simulink model "batteryModel"  (R2022b)
settings: Solver=VariableStepAuto  StartTime=0.0  StopTime=80000  RelTol=1e-3
PreLoadFcn:
  | first_run_this_to_import_nedc_data
  | batteryModel_ini
InitFcn:
  | first_run_this_to_import_nedc_data
  | batteryModel_ini
values from neighbouring files (symbols this model uses):
  Battery =     [BatteryParameters.mat]
  I = [1.29210780767e-28 1.29210780767e-28 1.29210780767e-28 1.29210780767e-28 1.29210780767e-28 1.29210780767e-28 1.29210780767e-28 1.29210780767e-28 1.29210780767e-28 1.29210780767e-28 1.29210780767e-28 4.77614030937 ... (41369 elements, 41369x1)]    [BatteryParameters.mat]
  OCVSOC = [2 2 0.95 1.1 0.95 0.79 1.02 0.92 0.75 0.87]    [BatteryParameters.mat]    (also in OCVSOC.mat)
  Ts = 1    [BatteryParameters.mat]    (also in myFunction.m; test1.m)
undefined symbols (not defined in the file or in its folder): sigbuilder_block
libraries: neural x50, fl_lib x7, nesl_utility x6, dspstat3 x3, simulink x2, sharedTrackingLibrary x2, batteryecm_lib x1, ctrlSharedLib x1
(part 1 of 3)
settings Model: Creator=The MathWorks, Inc.  LastModifiedBy=99661217
settings SolverCC: AlgebraicLoopSolver=TrustRegion
settings DataIOCC: SignalLogging=off  DSMLogging=off
settings OptimizationCC: DefaultParameterBehavior=Inlined  EnhancedBackFolding=on  PassReuseOutputArgsAs=Individual arguments  OptimizeBlockOrder=speed  DifferentSizesBufferReuse=on  OptimizationCustomize=off  EfficientTunableParamExpr=on
settings DebuggingCC: ParameterTunabilityLossMsg=error  UnconnectedInputMsg=warning  UnconnectedOutputMsg=warning  UnconnectedLineMsg=warning  PregeneratedLibrarySubsystemCodeDiagnostic=none  SFMachineParentedDataDiag=warning  ArithmeticOperatorsInVariantConditions=warning
settings ModelReferenceCC: EnableRefExpFcnMdlSchedulingChecks=on
settings SFSimCC: SimUseLocalCustomCode=off  MATLABDynamicMemAlloc=off  CustomCodeUndefinedFunction=UseInterfaceOnly
settings RTWCC: Description=Embedded Coder  SystemTargetFile=ert.tlc  GenCodeOnly=on  TemplateMakefile=ert_default_tmf  GenerateReport=on  RTWUseLocalCustomCode=off  IncludeHyperlinkInReport=on  LaunchReport=on  GenerateTraceInfo=on  GenerateTraceReport=on  GenerateTraceReportSl=on  GenerateTraceReportSf=on  GenerateTraceReportEml=on
settings CodeAppCC: ForceParamTrailComments=on  IgnoreCustomStorageClasses=off  OperatorAnnotations=on  SimulinkDataObjDesc=on  SFDataObjDesc=on  InsertBlockDesc=on
settings ERTTargetCC: TargetLangStandard=C99 (ISO)  GenerateSampleERTMain=on  InlinedParameterPlacement=NonHierarchical  ERTCustomFileTemplate=example_file_process.tlc
settings SimscapeCC: SimscapeNormalizeSystem=off

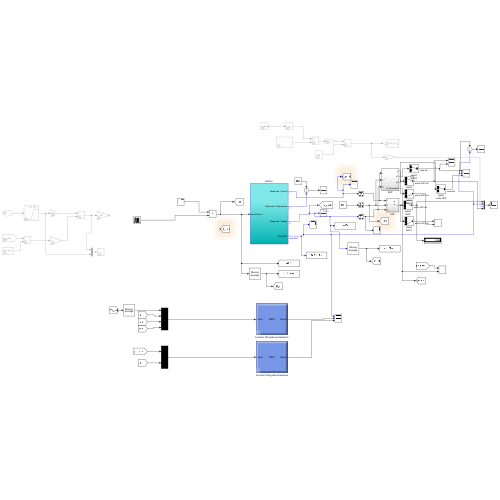
[thumbnail: Simulink's stored preview of the top-level diagram]
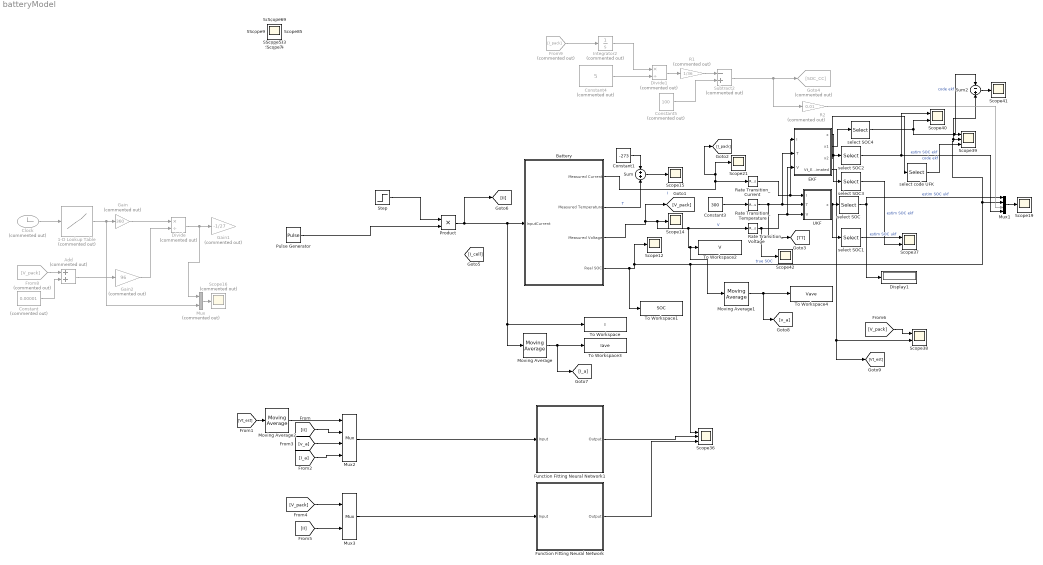
== system batteryModel ==
  1-D Lookup Table : Lookup_n-D  Commented=on  NumberOfTableDimensions=1  BreakpointsForDimension1=t  Table=I  InternalRulePriority=Speed  RndMeth=Simplest
  Add : Sum  Commented=on
  Battery : Subsystem
  Clock : Clock  Commented=on
  Constant : Constant  Commented=on  Value=0.00001
  Constant1 : Constant  Value=-273
  Constant3 : Constant  Value=300
  Constant4 : Constant  Commented=on  Value=5
  Constant5 : Constant  Commented=on  Value=100
  Display1 : Display
  Divide : Product  Commented=on  Inputs=*/
  Divide1 : Product  Commented=on  Inputs=*/
  EKF : Subsystem
  From8 : From  Commented=on  GotoTag=V_pack
  From9 : From  Commented=on  GotoTag=I_pack
  Function Fitting Neural Network : Subsystem
      mask help: Function Fitting Neural Network
      mask Display: e = 0.06;c1 = [120 150 230]/255;c2 = ([120 150 230]+0)/383;c3 = ([120 150 230]+128)/383;patch([0 1 1 0],[0 0 1 1],c1);patch([0 1 1 1-e 1-e 0+e],[0 0 1 1-e 0+e 0+e],c2);patch([0 0 1 1-e 0+e 0+e],[0 1 1 1-e 1-e 0+e],c3);plot([0 1 1 0 0],[0 0 1 1 0]);fprintf('NNET');port_label('input',1,' Input');port_label('output',1,'Output ');
  Function Fitting Neural Network1 : Subsystem
      mask help: Function Fitting Neural Network
      mask Display: e = 0.06;c1 = [120 150 230]/255;c2 = ([120 150 230]+0)/383;c3 = ([120 150 230]+128)/383;patch([0 1 1 0],[0 0 1 1],c1);patch([0 1 1 1-e 1-e 0+e],[0 0 1 1-e 0+e 0+e],c2);patch([0 0 1 1-e 0+e 0+e],[0 1 1 1-e 1-e 0+e],c3);plot([0 1 1 0 0],[0 0 1 1 0]);fprintf('NNET');port_label('input',1,' Input');port_label('output',1,'Output ');
  Gain : Gain  Commented=on  Gain=360
  Gain1 : Gain  Commented=on  Gain=-1/27
  Gain2 : Gain  Commented=on  Gain=96
  Goto4 : Goto  Commented=on  GotoTag=SOC_CC
  Integrator2 : Integrator  Commented=on
  Moving Average : dspstat3/Moving Average  Method=Sliding window  ForgettingFactorPort=off  SpecifyWindowLength=on  WindowLength=10  OverlapLength=9  AllowArbitraryInputLength=off  ForgettingFactor=0.9  SimulateUsing=Code generation
  Moving Average1 : dspstat3/Moving Average  Method=Sliding window  ForgettingFactorPort=off  SpecifyWindowLength=on  WindowLength=10  OverlapLength=9  AllowArbitraryInputLength=off  ForgettingFactor=0.9  SimulateUsing=Code generation
  Moving Average2 : dspstat3/Moving Average  Method=Sliding window  ForgettingFactorPort=off  SpecifyWindowLength=on  WindowLength=10  OverlapLength=9  AllowArbitraryInputLength=off  ForgettingFactor=0.9  SimulateUsing=Code generation
  Mux : Mux  Commented=on  Inputs=2
  Mux1 : Mux
  Mux2 : Mux
  Mux3 : Mux  Inputs=2
  Product : Product
  Pulse Generator : DiscretePulseGenerator  PulseType=Time based  Amplitude=-5  Period=60*60  PulseWidth=5/60*100
  R1 : Gain  Commented=on  Gain=1/36
  R2 : Gain  Commented=on  Gain=0.01
  Rate Transition_Current : RateTransition  OutPortSampleTime=Ts
  Rate Transition_Temperature : RateTransition  InitialCondition=300  OutPortSampleTime=Ts
  Rate Transition_Voltage : RateTransition  InitialCondition=4  OutPortSampleTime=Ts
  Scope{,1..15,17..35,41..42} (37 alike) : Scope
  Scope16 : Scope  Commented=on
  Scope36 : Scope  NumInputPorts=3
  Scope37 : Scope  NumInputPorts=2
  Scope38 : Scope  NumInputPorts=2
  Scope39 : Scope  NumInputPorts=3
  Scope40 : Scope  NumInputPorts=2
  Step : Step  SampleTime=0
  Subtract2 : Sum  Commented=on  Inputs=-+
  Sum : Sum
  Sum2 : Sum  Inputs=-+
  To Workspace : ToWorkspace  VariableName=I  SampleTime=-1
  To Workspace1 : ToWorkspace  VariableName=SOC  SampleTime=-1
  To Workspace2 : ToWorkspace  VariableName=V  SampleTime=-1
  To Workspace3 : ToWorkspace  VariableName=Iave  SampleTime=-1
  To Workspace4 : ToWorkspace  VariableName=Vave  SampleTime=-1
  UKF : Subsystem
  select SOC : Selector  InputPortWidth=5  IndexOptions=Index vector (dialog)  Indices=1  OutputSizes=1
  select SOC1 : Selector  InputPortWidth=5  IndexOptions=Index vector (dialog)  Indices=5  OutputSizes=1
  select SOC2 : Selector  InputPortWidth=5  IndexOptions=Index vector (dialog)  Indices=1  OutputSizes=1
  select SOC3 : Selector  InputPortWidth=5  IndexOptions=Index vector (dialog)  Indices=5  OutputSizes=1
  select SOC4 : Selector  InputPortWidth=2  IndexOptions=Index vector (dialog)  Indices=1  OutputSizes=1
  select code UFK : Selector  InputPortWidth=2  IndexOptions=Index vector (dialog)  Indices=1  OutputSizes=1
  wires:
  Battery/4(Real SOC) -> To Workspace1/1, Scope12/1, Sum2/2, Scope39/2, Mux1/2, Scope36/1  "true SOC"
  Divide/1 -> Gain1/1, Mux/1
  Battery/3(Measured Voltage) -> [V_pack], Moving Average1/1, To Workspace2/1, Rate Transition_Voltage/1, Scope14/1  "V"
  Battery/2(Measured Temperature) -> Sum/2  "T"
  Sum/1 -> Scope15/1
  Constant1/1 -> Sum/1
  From8/1 -> Add/1
  Clock/1 -> 1-D Lookup Table/1
  1-D Lookup Table/1 -> Mux/2, Gain/1
  Mux/1 -> Scope16/1
  Constant/1 -> Add/2
  Gain/1 -> Divide/1
  Add/1 -> Gain2/1
  Gain2/1 -> Divide/2
  Rate Transition_Temperature/1 -> [TT], UKF/2(T), EKF/2(T)
  Rate Transition_Voltage/1 -> Scope42/1, UKF/3(V), EKF/3(V)
  UKF/1(x) -> select SOC1/1, select SOC/1
  Rate Transition_Current/1 -> EKF/1(I), UKF/1(I)
  Battery/1(Measured Current) -> [I_pack], Scope21/1, Rate Transition_Current/1  "I"
  Mux1/1 -> Scope19/1
  select SOC/1 -> Mux1/1, Display1/1  "estim SOC ukf"
  Divide1/1 -> R1/1
  Integrator2/1 -> Divide1/1
  Constant5/1 -> Subtract2/2
  Constant4/1 -> Divide1/2
  R1/1 -> Subtract2/1
  Subtract2/1 -> R2/1, Goto4/1
  From9/1 -> Integrator2/1
  R2/1 -> Mux1/3
  Step/1 -> Product/1
  Product/1 -> [II], Moving Average/1, To Workspace/1, Battery/1(InputCurrent)
  select SOC1/1 -> Scope37/1  "estim SOC ukf"
  Constant3/1 -> Rate Transition_Temperature/1
  EKF/1(x) -> select SOC3/1, select SOC2/1
  select SOC2/1 -> Scope40/1, Mux1/4  "estim SOC ekf"
  select SOC3/1 -> Scope37/2  "estim SOC ekf"
  EKF/2(x1) -> select SOC4/1
  select SOC4/1 -> Sum2/1, Scope39/1, Scope40/2  "code ekf"
  Sum2/1 -> Scope41/1
  EKF/3(x2) -> select code UFK/1
  select code UFK/1 -> Scope39/3  "code ekf"
  Moving Average/1 -> [I_a], To Workspace3/1
  Moving Average1/1 -> [v_a], To Workspace4/1
  Function Fitting Neural Network1/1(Output) -> Scope36/2
  [Vt_est] -> Moving Average2/1
  [II] -> Mux2/2
  [v_a] -> Mux2/3
  [I_a] -> Mux2/4
  Mux2/1 -> Function Fitting Neural Network1/1(Input)
  Function Fitting Neural Network/1(Output) -> Scope36/3
  [V_pack] -> Mux3/1
  [II] -> Mux3/2
  Mux3/1 -> Function Fitting Neural Network/1(Input)
  [V_pack] -> Scope38/1
  EKF/4(Vt_Estimated) -> [Vt_est], Scope38/2
  Moving Average2/1 -> Mux2/1
  Pulse Generator/1 -> Product/2

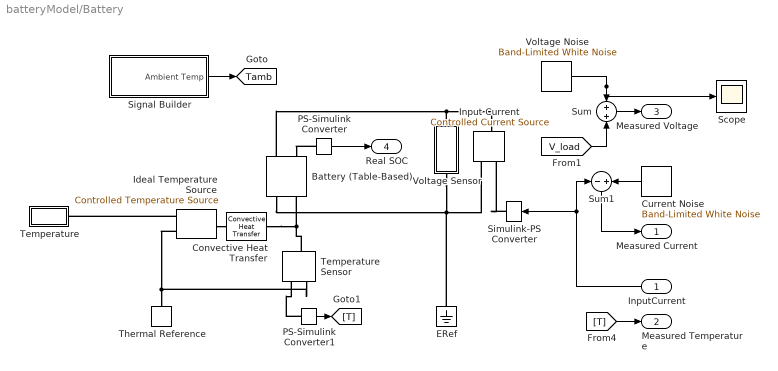
== system batteryModel/Battery ==
  InputCurrent : Inport
  Battery (Table-Based) : batteryecm_lib/Battery (Table-Based)  SOC_vec=Battery(1).SOC_LUT  T_dependence=simscape.enum.tablebattery.temperature_dependence.yes  prm_dir=simscape.enum.tablebattery.prm_dir.noCurrentDirectionality  T_vec=Battery(1).Temperature_LUT K  V0_mat=Battery(1).Em_LUT V  V0_vec=[3.1, 3.27, 3.31, 3.5] V  V_range=[0, inf] V  R0_mat=Battery(1).R0_LUT Ohm  R0_vec=[.015, .017, .012, .013] Ohm  R0_dis_mat=[.0117, .0085, .009; .011, .0085, .009; .0114, .0087, .0092; .0107, .0082, .0088; .0107, .0083, .0091; .0113, .0085, .0089; .0116, .0085, .0089] Ohm  R0_dis_vec=[.0085, .0085, .0087, .0082, .0083, .0085, .0085] Ohm  R0_ch_mat=[.0117, .0085, .009; .011, .0085, .009; .0114, .0087, .0092; .0107, .0082, .0088; .0107, .0083, .0091; .0113, .0085, .0089; .0116, .0085, .0089] Ohm  R0_ch_vec=[.0085, .0085, .0087, .0082, .0083, .0085, .0085] Ohm  AH=Battery(1).Capacity_LUT hr*A  prm_leak=simscape.enum.tablebattery.prm_leak.disabled  Rleak_vec=[8000, 7000, 6000] Ohm  Rleak=7e3 Ohm  extrapolation_option=simscape.enum.extrapolation.linear  SOC_port=simscape.enum.tablebattery.enable.yes  prm_dyn=simscape.enum.tablebattery.prm_dyn.rc3  R1_mat=Battery(1).R1_LUT Ohm  R1_vec=[.076, .022, .007, .043] Ohm  tau1_mat=Battery(1).t1_LUT s  tau1_vec=[148, 110, 27, 22] s  R2_mat=Battery(1).R2_LUT Ohm  R2_vec=[.382, .006, .007, .956] Ohm  tau2_mat=Battery(1).t2_LUT s  tau2_vec=[44, 24, 14, 13419] s  R3_mat=Battery(1).R3_LUT Ohm  R3_vec=[.382, .006, .007, .956] Ohm  tau3_mat=Battery(1).t3_LUT s  tau3_vec=[44, 24, 14, 13419] s  R4_mat=[.014, .382, .407; .028, .006, .007; .014, .007, .006; .333, .956, .912] Ohm  R4_vec=[.382, .006, .007, .956] Ohm  tau4_mat=[1, 44, 5644; 11, 24, 506; 2, 14, 330; 3310, 13419, 30216] s  tau4_vec=[44, 24, 14, 13419] s  R5_mat=[.014, .382, .407; .028, .006, .007; .014, .007, .006; .333, .956, .912] Ohm  R5_vec=[.382, .006, .007, .956] Ohm  tau5_mat=[1, 44, 5644; 11, 24, 506; 2, 14, 330; 3310, 13419, 30216] s  tau5_vec=[44, 24, 14, 13419] s  prm_fade=simscape.enum.tablebattery.prm_fade.equations  N0=100  dV0=0  dR0=0  dAH=0  dRleak=0  dR1=0  dR2=0  dR3=0  dR4=0  dR5=0  N0vec=[100, 200, 300]  Tfadevec=[298.15, 323.15] K  dV0vec=[0, 0, 0]  dR0vec=[0, 0, 0]  dAHvec=[0, 0, 0]  dRleakvec=[0, 0, 0]  dR1vec=[0, 0, 0]  dR2vec=[0, 0, 0]  dR3vec=[0, 0, 0]  dR4vec=[0, 0, 0]  dR5vec=[0, 0, 0]  dV0mat=[0, 0; 0, 0; 0, 0]  dR0mat=[0, 0; 0, 0; 0, 0]  dAHmat=[0, 0; 0, 0; 0, 0]  dRleakmat=[0, 0; 0, 0; 0, 0]  dR1mat=[0, 0; 0, 0; 0, 0]  dR2mat=[0, 0; 0, 0; 0, 0]  dR3mat=[0, 0; 0, 0; 0, 0]  dR4mat=[0, 0; 0, 0; 0, 0]  dR5mat=[0, 0; 0, 0; 0, 0]  prm_age_modeling=simscape.enum.tablebattery.prm_age_modeling.equation  storage_dt_age_vec=[0] d  storage_T_age_vec=[273] K  prm_age_OCV=simscape.enum.tablebattery.prm_age_OCV.OCV  OCV_age=0.9  SOC_age=0.6  prm_age_resistance=simscape.enum.tablebattery.prm_age.disabled  OCV_scaling_age_resistance=2.2134e6  OCV_offset_age_resistance=1.632e6  temp_exp_age_resistance=0.515833569 V  t_exp_age_resistance=0.75  T_age_vec_resistance=[273.15, 298.15, 323.15] K  dt_age_vec_resistance=[90, 180, 270, 360] d  dR0_age_vec=[0, 0, 0]  t_meas_dR0_age=100 d  dR0_age_mat=[0, 0, 0; 0, 0, 0; 0, 0, 0; 0, 0, 0]  prm_age_capacity=simscape.enum.tablebattery.prm_age.disabled  OCV_scaling_age_capacity=1.5097e07  OCV_offset_age_capacity=8.3625e06  temp_exp_age_capacity=0.6011 V  t_exp_age_capacity=0.75  T_age_vec_capacity=[273.15, 298.15, 323.15] K  dt_age_vec_capacity=[90, 180, 270, 360] d  dAH_age_vec=[0, 0, 0]  t_meas_dAH_age=100 d  dAH_age_mat=[0, 0, 0; 0, 0, 0; 0, 0, 0; 0, 0, 0]  thermal_port=simscape.enum.thermaleffects.model  temperature=Battery(1).T_init K  thermal_mass=Battery(1).cell_Cp_heat * Battery(1).cell_mass J/K  i_specify=off  i_priority=None  i=0 A  i_nominal_specify=off  i_nominal_unit=A  i_nominal_value=1  v_specify=off  v_priority=None  v=0 V  v_nominal_specify=off  v_nominal_unit=V  v_nominal_value=1  stateOfCharge_specify=on  stateOfCharge_priority=High  stateOfCharge=Battery(1).SOC0  stateOfCharge_nominal_specify=off  stateOfCharge_nominal_unit=1  stateOfCharge_nominal_value=1  num_cycles_specify=off  num_cycles_priority=High  num_cycles=0  num_cycles_nominal_specify=off  num_cycles_nominal_unit=1  num_cycles_nominal_value=1  cell_temperature_specify=off  cell_temperature_priority=High  cell_temperature=Battery(1).T_init K  cell_temperature_nominal_specify=off  cell_temperature_nominal_unit=K  cell_temperature_nominal_value=1
  Convective Heat Transfer : fl_lib/Thermal/Thermal Elements/Convective Heat Transfer  thermal_type=foundation.enum.constant_variable.constant  area=cell_area m^2  heat_tr_coeff=h_conv W/(m^2 * K)  min_heat_tr_coeff=1e-3 W/(K*m^2)  T_specify=off  T_priority=High  T=0 K  T_nominal_specify=off  T_nominal_unit=K  T_nominal_value=1  Q_specify=off  Q_priority=High  Q=0 J/s  Q_nominal_specify=off  Q_nominal_unit=J/s  Q_nominal_value=1
  Current Noise : simulink/Sources/Band-Limited White Noise  Cov=2.5e-2  Ts=Ts  seed=[1234]
  ERef : fl_lib/Electrical/Electrical Elements/Electrical Reference
  Ideal Temperature Source : fl_lib/Thermal/Thermal Sources/Controlled Temperature Source
  Input Current : fl_lib/Electrical/Electrical Sources/Controlled Current Source
  PS-Simulink Converter : nesl_utility/PS-Simulink Converter  PhysicalDomain=network_engine_domain  SubClassName=ps_output  LeftPortType=input  RightPortType=output  PseudoPeriodic=off  Frequencies=[]  VectorFormat=1-D array  Unit=inherit  AffineConversion=off
  PS-Simulink Converter1 : nesl_utility/PS-Simulink Converter  PhysicalDomain=network_engine_domain  SubClassName=ps_output  LeftPortType=input  RightPortType=output  PseudoPeriodic=off  Frequencies=[]  VectorFormat=1-D array  Unit=inherit  AffineConversion=off
  Scope : Scope
  Signal Builder : Subsystem  Tag=STV Subsys  LoadFcn=sigbuilder_block('load');  StartFcn=sigbuilder_block('start');  StopFcn=sigbuilder_block('stop');  ClipboardFcn=sigbuilder_block('clipboard');  mask(Sigbuilder block){tuvar=[0:10]}
      mask help: Simulink:masks:SigbuilderBlock_MD
      mask init:
      | if ~strcmp(get_param(bdroot(gcbh),'SimulationStatus'),'stopped') tuvar = sigbuilder_block('maskInit'); end
      settings: CopyFcn=sigbuilder_block('copy');  DeleteFcn=sigbuilder_block('delete');  ModelCloseFcn=sigbuilder_block('modelClose');  PreSaveFcn=sigbuilder_block('preSave');  PauseFcn=sigbuilder_block('pause');  ContinueFcn=sigbuilder_block('continue');  NameChangeFcn=sigbuilder_block('namechange');  OpenFcn=sigbuilder_block('open',[45.6 240 978 346.2 ]);  CloseFcn=sigbuilder_block('close');
      mask Display: plot(0, 0, 100, 100,[2, 2, 32, 32, 2], [68, 8, 8, 68, 68],[32, 2], [38, 38], [32, 19, 2],[53, 60, 44], [32, 17, 17, 2],[16, 16, 31, 31]);txt = getActiveGroup(gcbh);text(2, 100, txt,'verticalAlignment', 'top');
  Simulink-PS Converter : nesl_utility/Simulink-PS Converter  PhysicalDomain=network_engine_domain  SubClassName=ps_input  LeftPortType=input  RightPortType=output  PseudoPeriodic=off  Frequencies=[]  NoiseDistribution=none  NoiseParameters=[]  Unit=A  AffineConversion=off  FilteringAndDerivatives=zero  SimscapeFilterOrder=1  InputFilterTimeConstant=.001  UdotUserProvided=1
  Sum : Sum
  Sum1 : Sum  Inputs=-+
  Temperature : Subsystem
      mask Display: disp('Tamb')
  Temperature Sensor : fl_lib/Thermal/Thermal Sensors/Temperature Sensor
  Thermal Reference : fl_lib/Thermal/Thermal Elements/Thermal Reference
  Voltage Sensor : Subsystem
      mask Display: disp('V_load')
  Voltage Noise : simulink/Sources/Band-Limited White Noise  Cov=0.5e-3  Ts=Ts  seed=[1234]
  Measured Current : Outport  VectorParamsAs1DForOutWhenUnconnected=off
  Measured Temperature : Outport  Port=2  VectorParamsAs1DForOutWhenUnconnected=off
  Measured Voltage : Outport  Port=3  VectorParamsAs1DForOutWhenUnconnected=off
  Real SOC : Outport  Port=4  VectorParamsAs1DForOutWhenUnconnected=off
  tag scope: Tamb=global
  wires:
  Signal Builder/1(Ambient Temp) -> [Tamb]
  [V_load] -> Sum/2
  Sum/1 -> Measured Voltage/1
  Sum1/1 -> Measured Current/1
  InputCurrent/1 -> Sum1/1, Simulink-PS Converter/1
  [T] -> Measured Temperature/1
  PS-Simulink Converter/1 -> Real SOC/1
  PS-Simulink Converter1/1 -> [T]
  Voltage Noise/1 -> Scope/1, Sum/1
  Current Noise/1 -> Sum1/2
  connections:
  Convective Heat Transfer/RConn1 -- Battery (Table-Based)/RConn2 -- Temperature Sensor/LConn1
  Voltage Sensor/RConn1 -- Input Current/RConn2 -- ERef/LConn1 -- Battery (Table-Based)/RConn1
  Battery (Table-Based)/LConn1 -- Input Current/LConn1 -- Voltage Sensor/LConn1
  Ideal Temperature Source/RConn1 -- Temperature/LConn1
  Ideal Temperature Source/RConn2 -- Thermal Reference/LConn1 -- Temperature Sensor/RConn1
  Simulink-PS Converter/RConn1 -- Input Current/RConn1
  Ideal Temperature Source/LConn1 -- Convective Heat Transfer/LConn1
  PS-Simulink Converter/LConn1 -- Battery (Table-Based)/LConn2
  PS-Simulink Converter1/LConn1 -- Temperature Sensor/RConn2

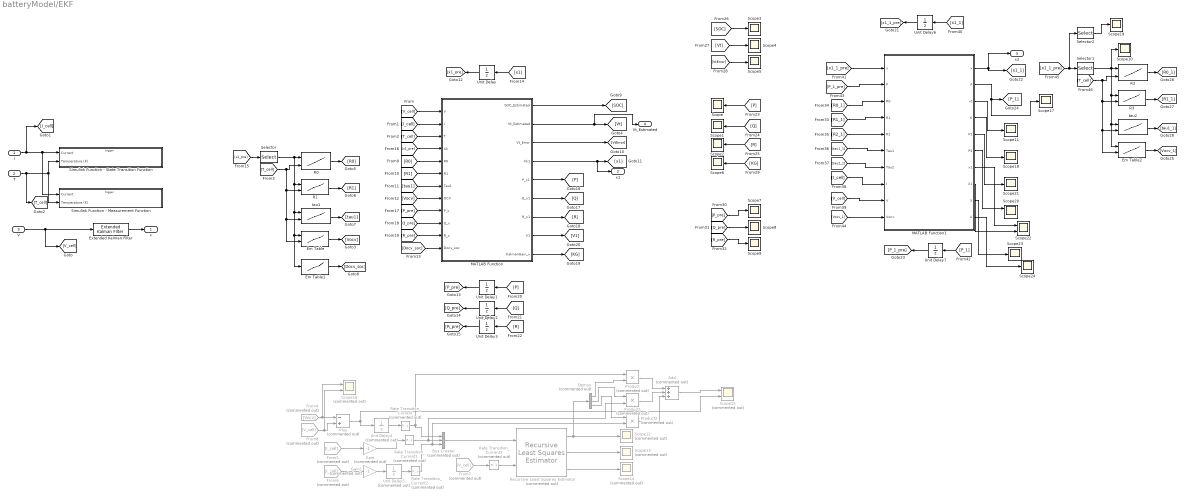
== system batteryModel/EKF ==
  I : Inport
  T : Inport  Port=2
  V : Inport  Port=3
  Add : Sum  Commented=on  Inputs=+++
  Bus Creator : BusCreator  Commented=on  Inputs=3
  Demux : Demux  Commented=on  Outputs=3
  Em Table : Lookup_n-D  BreakpointsForDimension1=Battery.SOC_LUT  BreakpointsForDimension2=Battery.Temperature_LUT  Table=Battery.Em_LUT  InternalRulePriority=Speed  RndMeth=Simplest
      settings: InputPortMap=u0,u1
  Em Table1 : Lookup_n-D  NumberOfTableDimensions=1  BreakpointsForDimension1=Battery.SOC_LUT  BreakpointsForDimension2=Battery.Temperature_LUT  Table=OCVSOC  InternalRulePriority=Speed  RndMeth=Simplest
  Em Table2 : Lookup_n-D  BreakpointsForDimension1=Battery.SOC_LUT  BreakpointsForDimension2=Battery.Temperature_LUT  Table=Battery.Em_LUT  InternalRulePriority=Speed  RndMeth=Simplest
      settings: InputPortMap=u0,u1
  Extended Kalman Filter : sharedTrackingLibrary/Extended Kalman Filter  StateTransitionFcn=batteryStateFcn1  HasStateTransitionJacobianFcn=off  HasAdditiveProcessNoise=Additive  ProcessNoise=1e-10*eye(5)  HasTimeVaryingProcessNoise=off  HasStateTransitionFcnExtraArgument=0  InitialState=[0.1; 0; 0; 0; 0]  InitialStateCovariance=[2000 1 1 1 1]  MeasurementFcn1=batteryMeasurementFcn1  HasMeasurementJacobianFcn1=off  HasMeasurementEnablePort1=off  HasAdditiveMeasurementNoise1=Additive  MeasurementNoise1=50  HasTimeVaryingMeasurementNoise1=off  HasMeasurementFcnExtraArgument1=0  HasMeasurementWrapping1=off  MeasurementFcn2=myMeasurementFcn  HasMeasurementJacobianFcn2=off  HasMeasurementEnablePort2=off  HasAdditiveMeasurementNoise2=Additive  MeasurementNoise2=1  HasTimeVaryingMeasurementNoise2=off  HasMeasurementFcnExtraArgument2=0  HasMeasurementWrapping2=off  MeasurementFcn3=myMeasurementFcn  HasMeasurementJacobianFcn3=off  HasMeasurementEnablePort3=off  HasAdditiveMeasurementNoise3=Additive  MeasurementNoise3=1  HasTimeVaryingMeasurementNoise3=off  HasMeasurementFcnExtraArgument3=0  HasMeasurementWrapping3=off  MeasurementFcn4=myMeasurementFcn  HasMeasurementJacobianFcn4=off  HasMeasurementEnablePort4=off  HasAdditiveMeasurementNoise4=Additive  MeasurementNoise4=1  HasTimeVaryingMeasurementNoise4=off  HasMeasurementFcnExtraArgument4=0  HasMeasurementWrapping4=off  MeasurementFcn5=myMeasurementFcn  HasMeasurementJacobianFcn5=off  HasMeasurementEnablePort5=off  HasAdditiveMeasurementNoise5=Additive  MeasurementNoise5=1  HasTimeVaryingMeasurementNoise5=off  HasMeasurementFcnExtraArgument5=0  HasMeasurementWrapping5=off  EnableMultirate=off  StateTransitionFcnSampleTime=1  MeasurementFcn1SampleTime=1  MeasurementFcn2SampleTime=1  MeasurementFcn3SampleTime=1  MeasurementFcn4SampleTime=1  MeasurementFcn5SampleTime=1  UseCurrentEstimator=off  OutputStateCovariance=off  DataType=double  SampleTime=Ts  NumberOfMeasurements=1
  From4 : From  Commented=on  GotoTag=Vocv
  From5 : From  Commented=on  GotoTag=I_cell
  From6 : From  Commented=on  GotoTag=I_cell
  From7 : From  Commented=on  GotoTag=V_cell
  From8 : From  Commented=on  GotoTag=V_cell
  Gain : Gain  Commented=on  Gain=-1
  Gain1 : Gain  Commented=on  Gain=-1
  MATLAB Function : MATLAB Function  TreatAsAtomicUnit=on
  MATLAB Function1 : MATLAB Function  TreatAsAtomicUnit=on  SystemSampleTime=Ts
  Plus : Sum  Commented=on  Inputs=-+
  Product : Product  Commented=on
  Product1 : Product  Commented=on
  Product2 : Product  Commented=on
  R0 : Lookup_n-D  BreakpointsForDimension1=Battery.SOC_LUT  BreakpointsForDimension2=Battery.Temperature_LUT  Table=Battery.R0_LUT  InternalRulePriority=Speed  RndMeth=Simplest
      settings: InputPortMap=u0,u1
  R1 : Lookup_n-D  BreakpointsForDimension1=Battery.SOC_LUT  BreakpointsForDimension2=Battery.Temperature_LUT  Table=Battery.R1_LUT  InternalRulePriority=Speed  RndMeth=Simplest
      settings: InputPortMap=u0,u1
  R2 : Lookup_n-D  BreakpointsForDimension1=Battery.SOC_LUT  BreakpointsForDimension2=Battery.Temperature_LUT  Table=Battery.R0_LUT  InternalRulePriority=Speed  RndMeth=Simplest
      settings: InputPortMap=u0,u1
  R3 : Lookup_n-D  BreakpointsForDimension1=Battery.SOC_LUT  BreakpointsForDimension2=Battery.Temperature_LUT  Table=Battery.R1_LUT  InternalRulePriority=Speed  RndMeth=Simplest
      settings: InputPortMap=u0,u1
  Rate Transition_Current{,1..3} (4 alike) : RateTransition  Commented=on  OutPortSampleTime=2*Ts
  Recursive Least Squares Estimator : ctrlSharedLib/Recursive Least Squares Estimator  Commented=on  InitialEstimateSource=None  InitialParameterData=3  P0=[1000 0 0;0 1000 0;0 0 1000]  InitialRegressors=0  InitialOutputs=0  History=Infinite  WindowLength=300  EstimationMethod=Forgetting Factor  AdaptationParameter=0.98  HasTimeVaryingAdaptationParameter=off  NormalizationBias=eps  OutputError=on  OutputP=on  AddEnablePort=off  InputProcessing=Sample-based  Ts=2*Ts
      settings: LibrarySourceBlock=slident/Estimators/Recursive Least Squares Estimator
  Scope{,1..11,17..19,21,23..24} (18 alike) : Scope
  Scope12 : Scope  Commented=on
  Scope13 : Scope  Commented=on
  Scope14 : Scope  Commented=on
  Scope15 : Scope  Commented=on  NumInputPorts=2
  Scope16 : Scope  Commented=on  NumInputPorts=2
  Scope20 : Scope  NumInputPorts=2
  Scope22 : Scope  NumInputPorts=2
  Selector : Selector  InputPortWidth=2  IndexOptions=Index vector (dialog)  Indices=[1]  OutputSizes=1
  Selector1 : Selector  InputPortWidth=2  IndexOptions=Index vector (dialog)  Indices=[1]  OutputSizes=1
  Selector2 : Selector  InputPortWidth=2  IndexOptions=Index vector (dialog)  Indices=[2]  OutputSizes=1
  Simulink Function - Measurement Function : Subsystem  TreatAsAtomicUnit=on
  Simulink Function - State Transition Function : Subsystem  TreatAsAtomicUnit=on
  Unit Delay : UnitDelay  InitialCondition=[1 0]  SampleTime=Ts  HasFrameUpgradeWarning=on
  Unit Delay1 : UnitDelay  InitialCondition=[200 0 ;0 1]  SampleTime=Ts  HasFrameUpgradeWarning=on
  Unit Delay2 : UnitDelay  InitialCondition=[1.0e-10 0 ;0 1.0e-10]  SampleTime=Ts  HasFrameUpgradeWarning=on
  Unit Delay3 : UnitDelay  InitialCondition=50  SampleTime=Ts  HasFrameUpgradeWarning=on
  Unit Delay4 : UnitDelay  Commented=on  SampleTime=Ts  HasFrameUpgradeWarning=on
  Unit Delay5 : UnitDelay  Commented=on  SampleTime=Ts  HasFrameUpgradeWarning=on
  Unit Delay6 : UnitDelay  InitialCondition=[1 0]  SampleTime=Ts  HasFrameUpgradeWarning=on
  Unit Delay7 : UnitDelay  InitialCondition=[1 0 ;0 1]  SampleTime=Ts  HasFrameUpgradeWarning=on
  tau1 : Lookup_n-D  BreakpointsForDimension1=Battery.SOC_LUT  BreakpointsForDimension2=Battery.Temperature_LUT  Table=Battery.t1_LUT  InternalRulePriority=Speed  RndMeth=Simplest
      settings: InputPortMap=u0,u1
  tau2 : Lookup_n-D  BreakpointsForDimension1=Battery.SOC_LUT  BreakpointsForDimension2=Battery.Temperature_LUT  Table=Battery.t1_LUT  InternalRulePriority=Speed  RndMeth=Simplest
      settings: InputPortMap=u0,u1
  x : Outport  VectorParamsAs1DForOutWhenUnconnected=off
  x1 : Outport  Port=2  VectorParamsAs1DForOutWhenUnconnected=off
  x2 : Outport  Port=3  VectorParamsAs1DForOutWhenUnconnected=off
  Vt_Estimated : Outport  Port=4
  wires:
  V/1 -> [V_cell], Extended Kalman Filter/1
  T/1 -> [T_cell], Simulink Function - Measurement Function/2(Temperature (K)), Simulink Function - State Transition Function/2(Temperature (K))
  I/1 -> [I_cell], Simulink Function - Measurement Function/1(Current), Simulink Function - State Transition Function/1(Current)
  Extended Kalman Filter/1 -> x/1
  MATLAB Function/4(Xk1) -> [x1], x1/1
  [V_cell] -> MATLAB Function/1(V)
  [I_cell] -> MATLAB Function/2(I)
  [T_cell] -> MATLAB Function/3(T)
  Selector/1 -> Em Table1/1, Em Table/1, tau1/1, R1/1, R0/1
  [T_cell] -> Em Table/2, tau1/2, R1/2, R0/2
  Em Table/1 -> [Vocv]
  MATLAB Function/1(SOC_Estimated) -> [SOC]
  From6/1 -> Gain1/1
  Unit Delay4/1 -> Rate Transition_Current/1
  From5/1 -> Gain/1
  Unit Delay5/1 -> Rate Transition_Current2/1
  Bus Creator/1 -> Recursive Least Squares Estimator/1
  From7/1 -> Rate Transition_Current3/1
  Recursive Least Squares Estimator/1 -> Demux/1, Scope12/1
  From4/1 -> Scope16/1, Plus/1
  From8/1 -> Scope16/2, Plus/2
  Plus/1 -> Scope15/2, Unit Delay4/1
  Gain/1 -> Rate Transition_Current1/1
  Gain1/1 -> Unit Delay5/1
  Recursive Least Squares Estimator/2 -> Scope13/1
  Recursive Least Squares Estimator/3 -> Scope14/1
  Demux/1 -> Product/2
  Demux/2 -> Product1/1
  Demux/3 -> Product2/1
  Product/1 -> Add/1
  Product1/1 -> Add/2
  Product2/1 -> Add/3
  Add/1 -> Scope15/1
  Rate Transition_Current/1 -> Product/1, Bus Creator/1
  Rate Transition_Current1/1 -> Product1/2, Bus Creator/2
  Rate Transition_Current2/1 -> Product2/2, Bus Creator/3
  Rate Transition_Current3/1 -> Recursive Least Squares Estimator/2
  R0/1 -> [R0]
  [R0] -> MATLAB Function/5(R0)
  R1/1 -> [R1]
  [R1] -> MATLAB Function/6(R1)
  tau1/1 -> [tau1]
  [tau1] -> MATLAB Function/7(Tau1)
  Em Table1/1 -> [Docv_soc]
  [Vocv] -> MATLAB Function/8(OCV)
  [Docv_soc] -> MATLAB Function/12(Docv_soc)
  MATLAB Function/2(Vt_Estimated) -> Vt_Estimated/1, [Vt]
  MATLAB Function/3(Vt_Error) -> [VtError]
  [x1] -> Unit Delay/1
  Unit Delay/1 -> [x1_pre]
  [x1_pre] -> Selector/1
  [x1_pre] -> MATLAB Function/4(Xk)
  [P_pre] -> MATLAB Function/9(P_x)
  [Q_pre] -> MATLAB Function/10(Q_x)
  [R_pre] -> MATLAB Function/11(R_x)
  Unit Delay1/1 -> [P_pre]
  Unit Delay2/1 -> [Q_pre]
  Unit Delay3/1 -> [R_pre]
  MATLAB Function/5(P_x1) -> [P]
  MATLAB Function/6(Q_x1) -> [Q]
  MATLAB Function/7(R_x1) -> [R]
  MATLAB Function/9(KalmanGain_x) -> [KG]
  [P] -> Unit Delay1/1
  [Q] -> Unit Delay2/1
  [R] -> Unit Delay3/1
  MATLAB Function/8(V1) -> [V1]
  [P] -> Scope/1
  [Q] -> Scope1/1
  [R] -> Scope2/1
  [SOC] -> Scope3/1
  [Vt] -> Scope4/1
  [VtError] -> Scope5/1
  [KG] -> Scope6/1
  [P_pre] -> Scope7/1
  [Q_pre] -> Scope8/1
  [R_pre] -> Scope9/1
  [R2_1] -> MATLAB Function1/5(R2)
  [R1_1] -> MATLAB Function1/4(R1)
  [R0_1] -> MATLAB Function1/3(R0)
  [tau1_1] -> MATLAB Function1/6(Tau1)
  [tau2_1] -> MATLAB Function1/7(Tau2)
  [I_cell] -> MATLAB Function1/8(I)
  [V_cell] -> MATLAB Function1/9(V)
  Unit Delay6/1 -> [x1_1_pre]
  [x1_1] -> Unit Delay6/1
  MATLAB Function1/1(x) -> [x1_1], x2/1
  [x1_1_pre] -> MATLAB Function1/1("x ")
  Unit Delay7/1 -> [P_1_pre]
  [P_1] -> Unit Delay7/1
  MATLAB Function1/2(P) -> Scope17/1, [P_1]
  [P_1_pre] -> MATLAB Function1/2("P ")
  [Vocv_1] -> MATLAB Function1/10(Vocv)
  [x1_1_pre] -> Selector2/1, Selector1/1
  tau2/1 -> [tau1_1]
  R3/1 -> [R1_1]
  R2/1 -> [R0_1]
  Em Table2/1 -> [Vocv_1]
  [T_cell] -> R2/2, R3/2, tau2/2, Em Table2/2
  Selector1/1 -> Scope10/1, R2/1, R3/1, tau2/1, Em Table2/1
  MATLAB Function1/3(vt) -> Scope11/1
  MATLAB Function1/4(K) -> Scope18/1
  Selector2/1 -> Scope19/1
  MATLAB Function1/6(P2) -> Scope20/1
  MATLAB Function1/5(P1) -> Scope21/1
  MATLAB Function1/7(x1) -> Scope22/1
  MATLAB Function1/8(X1) -> Scope22/2
  MATLAB Function1/9(X) -> Scope23/1
  MATLAB Function1/10(A) -> Scope24/1

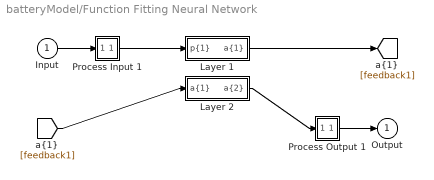
== system batteryModel/Function Fitting Neural Network ==
  Input : Inport  PortDimensions=2
      mask Display: e = 0.06;c1 = [120 230 180]/255;c2 = ([120 230 180]+0)/(256+128);c3 = ([120 230 180]+128)/(256+128);patch([0 1 1 0],[0 0 1 1],c1);patch([0 1 1 1-e 1-e 0+e],[0 0 1 1-e 0+e 0+e],c2);patch([0 0 1 1-e 0+e 0+e],[0 1 1 1-e 1-e 0+e],c3);plot([0 1 1 0 0],[0 0 1 1 0]);
  Layer 1 : Subsystem
      mask Display: e = 0.06;c1 = [120 150 230]/255;c2 = ([120 150 230]+0)/383;c3 = ([120 150 230]+128)/383;patch([0 1 1 0],[0 0 1 1],c1);patch([0 1 1 1-e 1-e 0+e],[0 0 1 1-e 0+e 0+e],c2);patch([0 0 1 1-e 0+e 0+e],[0 1 1 1-e 1-e 0+e],c3);plot([0 1 1 0 0],[0 0 1 1 0]);
  Layer 2 : Subsystem
      mask Display: e = 0.06;c1 = [120 150 230]/255;c2 = ([120 150 230]+0)/383;c3 = ([120 150 230]+128)/383;patch([0 1 1 0],[0 0 1 1],c1);patch([0 1 1 1-e 1-e 0+e],[0 0 1 1-e 0+e 0+e],c2);patch([0 0 1 1-e 0+e 0+e],[0 1 1 1-e 1-e 0+e],c3);plot([0 1 1 0 0],[0 0 1 1 0]);
  Process Input 1 : Subsystem
      mask Display: e = 0.06;c1 = [120 150 230]/255;c2 = ([120 150 230]+0)/383;c3 = ([120 150 230]+128)/383;patch([0 1 1 0],[0 0 1 1],c1);patch([0 1 1 1-e 1-e 0+e],[0 0 1 1-e 0+e 0+e],c2);patch([0 0 1 1-e 0+e 0+e],[0 1 1 1-e 1-e 0+e],c3);plot([0 1 1 0 0],[0 0 1 1 0]);
  Process Output 1 : Subsystem
      mask Display: e = 0.06;c1 = [120 150 230]/255;c2 = ([120 150 230]+0)/383;c3 = ([120 150 230]+128)/383;patch([0 1 1 0],[0 0 1 1],c1);patch([0 1 1 1-e 1-e 0+e],[0 0 1 1-e 0+e 0+e],c2);patch([0 0 1 1-e 0+e 0+e],[0 1 1 1-e 1-e 0+e],c3);plot([0 1 1 0 0],[0 0 1 1 0]);
  Output : Outport  InitialOutput=0
      mask Display: e = 0.06;c1 = [120 230 180]/255;c2 = ([120 230 180]+0)/(256+128);c3 = ([120 230 180]+128)/(256+128);patch([0 1 1 0],[0 0 1 1],c1);patch([0 1 1 1-e 1-e 0+e],[0 0 1 1-e 0+e 0+e],c2);patch([0 0 1 1-e 0+e 0+e],[0 1 1 1-e 1-e 0+e],c3);plot([0 1 1 0 0],[0 0 1 1 0]);
  wires:
  Input/1 -> Process Input 1/1(x)
  Process Output 1/1(y) -> Output/1
  Process Input 1/1(p) -> Layer 1/1("p{1}")
  Layer 1/1("a{1}") -> [feedback1]
  [feedback1] -> Layer 2/1("a{1} ")
  Layer 2/1("a{2}") -> Process Output 1/1(a)

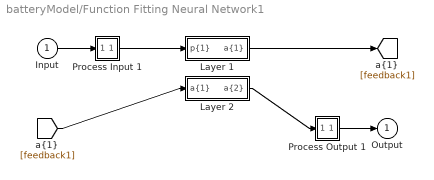
== system batteryModel/Function Fitting Neural Network1 ==
  Input : Inport  PortDimensions=4
      mask Display: e = 0.06;c1 = [120 230 180]/255;c2 = ([120 230 180]+0)/(256+128);c3 = ([120 230 180]+128)/(256+128);patch([0 1 1 0],[0 0 1 1],c1);patch([0 1 1 1-e 1-e 0+e],[0 0 1 1-e 0+e 0+e],c2);patch([0 0 1 1-e 0+e 0+e],[0 1 1 1-e 1-e 0+e],c3);plot([0 1 1 0 0],[0 0 1 1 0]);
  Layer 1 : Subsystem
      mask Display: e = 0.06;c1 = [120 150 230]/255;c2 = ([120 150 230]+0)/383;c3 = ([120 150 230]+128)/383;patch([0 1 1 0],[0 0 1 1],c1);patch([0 1 1 1-e 1-e 0+e],[0 0 1 1-e 0+e 0+e],c2);patch([0 0 1 1-e 0+e 0+e],[0 1 1 1-e 1-e 0+e],c3);plot([0 1 1 0 0],[0 0 1 1 0]);
  Layer 2 : Subsystem
      mask Display: e = 0.06;c1 = [120 150 230]/255;c2 = ([120 150 230]+0)/383;c3 = ([120 150 230]+128)/383;patch([0 1 1 0],[0 0 1 1],c1);patch([0 1 1 1-e 1-e 0+e],[0 0 1 1-e 0+e 0+e],c2);patch([0 0 1 1-e 0+e 0+e],[0 1 1 1-e 1-e 0+e],c3);plot([0 1 1 0 0],[0 0 1 1 0]);
  Process Input 1 : Subsystem
      mask Display: e = 0.06;c1 = [120 150 230]/255;c2 = ([120 150 230]+0)/383;c3 = ([120 150 230]+128)/383;patch([0 1 1 0],[0 0 1 1],c1);patch([0 1 1 1-e 1-e 0+e],[0 0 1 1-e 0+e 0+e],c2);patch([0 0 1 1-e 0+e 0+e],[0 1 1 1-e 1-e 0+e],c3);plot([0 1 1 0 0],[0 0 1 1 0]);
  Process Output 1 : Subsystem
      mask Display: e = 0.06;c1 = [120 150 230]/255;c2 = ([120 150 230]+0)/383;c3 = ([120 150 230]+128)/383;patch([0 1 1 0],[0 0 1 1],c1);patch([0 1 1 1-e 1-e 0+e],[0 0 1 1-e 0+e 0+e],c2);patch([0 0 1 1-e 0+e 0+e],[0 1 1 1-e 1-e 0+e],c3);plot([0 1 1 0 0],[0 0 1 1 0]);
  Output : Outport  InitialOutput=0
      mask Display: e = 0.06;c1 = [120 230 180]/255;c2 = ([120 230 180]+0)/(256+128);c3 = ([120 230 180]+128)/(256+128);patch([0 1 1 0],[0 0 1 1],c1);patch([0 1 1 1-e 1-e 0+e],[0 0 1 1-e 0+e 0+e],c2);patch([0 0 1 1-e 0+e 0+e],[0 1 1 1-e 1-e 0+e],c3);plot([0 1 1 0 0],[0 0 1 1 0]);
  wires:
  Input/1 -> Process Input 1/1(x)
  Process Output 1/1(y) -> Output/1
  Process Input 1/1(p) -> Layer 1/1("p{1}")
  Layer 1/1("a{1}") -> [feedback1]
  [feedback1] -> Layer 2/1("a{1} ")
  Layer 2/1("a{2}") -> Process Output 1/1(a)

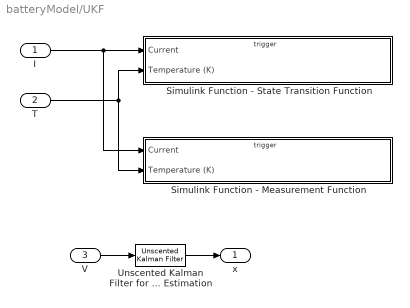
== system batteryModel/UKF ==
  I : Inport
  T : Inport  Port=2
  V : Inport  Port=3
  Simulink Function - Measurement Function : Subsystem  TreatAsAtomicUnit=on
  Simulink Function - State Transition Function : Subsystem  TreatAsAtomicUnit=on
  Unscented Kalman Filter for SOC Estimation : sharedTrackingLibrary/Unscented Kalman Filter  StateTransitionFcn=batteryStateFcn  HasAdditiveProcessNoise=Additive  ProcessNoise=1e-10*eye(5)  HasTimeVaryingProcessNoise=off  HasStateTransitionFcnExtraArgument=0  InitialState=[0.1; 0; 0; 0; 0]  InitialStateCovariance=[2000 1 1 1 1]  Alpha=1  Beta=2  Kappa=0  MeasurementFcn1=batteryMeasurementFcn  HasMeasurementEnablePort1=off  HasAdditiveMeasurementNoise1=Additive  MeasurementNoise1=10  HasTimeVaryingMeasurementNoise1=off  HasMeasurementFcnExtraArgument1=0  HasMeasurementWrapping1=off  MeasurementFcn2=myMeasurementFcn  HasMeasurementEnablePort2=off  HasAdditiveMeasurementNoise2=Additive  MeasurementNoise2=1  HasTimeVaryingMeasurementNoise2=off  HasMeasurementFcnExtraArgument2=0  HasMeasurementWrapping2=off  MeasurementFcn3=myMeasurementFcn  HasMeasurementEnablePort3=off  HasAdditiveMeasurementNoise3=Additive  MeasurementNoise3=1  HasTimeVaryingMeasurementNoise3=off  HasMeasurementFcnExtraArgument3=0  HasMeasurementWrapping3=off  MeasurementFcn4=myMeasurementFcn  HasMeasurementEnablePort4=off  HasAdditiveMeasurementNoise4=Additive  MeasurementNoise4=1  HasTimeVaryingMeasurementNoise4=off  HasMeasurementFcnExtraArgument4=0  HasMeasurementWrapping4=off  MeasurementFcn5=myMeasurementFcn  HasMeasurementEnablePort5=off  HasAdditiveMeasurementNoise5=Additive  MeasurementNoise5=1  HasTimeVaryingMeasurementNoise5=off  HasMeasurementFcnExtraArgument5=0  HasMeasurementWrapping5=off  EnableMultirate=off  StateTransitionFcnSampleTime=-1  MeasurementFcn1SampleTime=-1  MeasurementFcn2SampleTime=-1  MeasurementFcn3SampleTime=-1  MeasurementFcn4SampleTime=-1  MeasurementFcn5SampleTime=-1  UseCurrentEstimator=on  OutputStateCovariance=off  DataType=double  SampleTime=Ts  NumberOfMeasurements=1
  x : Outport  VectorParamsAs1DForOutWhenUnconnected=off
  wires:
  T/1 -> Simulink Function - Measurement Function/2(Temperature (K)), Simulink Function - State Transition Function/2(Temperature (K))
  V/1 -> Unscented Kalman Filter for SOC Estimation/1
  I/1 -> Simulink Function - Measurement Function/1(Current), Simulink Function - State Transition Function/1(Current)
  Unscented Kalman Filter for SOC Estimation/1 -> x/1

== system batteryModel/Battery/Signal Builder ==
  Demux : Demux  Tag=STV Demux  Outputs=1
      settings: DisplayOption=none
  FromWs : FromWorkspace  Tag=STV FromWs  VariableName=tuvar
      SigBuilderData=|
      | common.afterFinalStr = 'Extrapolate'
      | common.sampleTime = 0
      | dataSet(1).timeRange = [0 40000]
      | dataSet(1).name = 'Pulse'
      | dataSet(2).timeRange = [0 40000]
      | dataSet(2).name = 'Constant'
      | sbobj.Name = 'Signal Builder'
      | sbobj.Groups(1).Name = 'Pulse'
      | sbobj.Groups(1).Signals.Name = 'Ambient Temp'
      | sbobj.Groups(1).Signals.XData = [0 300 2100 3600 3960 7200 7560 10800 11160 14400 14760 18000 18360 21600 21960 25200 25560 28800 29160 32400 32760 36000 36360 40000]
      | sbobj.Groups(1).Signals.YData = [20 20 20 20 20 20 20 20 20 20 20 20 20 20 20 20 20 20 20 20 20 20 20 20]
      | sbobj.Groups(1).TimeRange = [0 40000]
      | sbobj.Groups(2).Name = 'Constant'
      | sbobj.Groups(2).Signals.Name = 'Ambient Temp'
      | sbobj.Groups(2).Signals.XData = [0 360 9100 11800 28200 33800 40000]
      | sbobj.Groups(2).Signals.YData = [20 20.09 22.275 22.95 27.05 28.45 30]
      | sbobj.Groups(2).TimeRange = [0 40000]
  Ambient Temp : Outport  Tag=STV Outport  VectorParamsAs1DForOutWhenUnconnected=off
  wires:
  FromWs/1 -> Demux/1
  Demux/1 -> Ambient Temp/1

== system batteryModel/Battery/Temperature ==
  Simulink-PS Converter1 : nesl_utility/Simulink-PS Converter  PhysicalDomain=network_engine_domain  SubClassName=ps_input  LeftPortType=input  RightPortType=output  PseudoPeriodic=off  Frequencies=[]  NoiseDistribution=none  NoiseParameters=[]  Unit=degC  AffineConversion=on  FilteringAndDerivatives=zero  SimscapeFilterOrder=1  InputFilterTimeConstant=.001  UdotUserProvided=1
  Solver Configuration : nesl_utility/Solver Configuration  PhysicalDomain=network_engine_domain  SubClassName=solver  LeftPortType=input  RightPortType=generic  Tones=[]  Harmonics=[]  SimulateNoise=off  Profile=off  UseLocalSampling=off  EnableSwitchedLinearOptims=on  FrequencyDomain=off  UseCCode=off  RelTol=0.001  AbsTol=1e-06  MinStep=1e-09  ToWorkspace=off  RevertToSquareIcSolve=off  NumHomotopyIterations=100  PhasorMode=off  PhasorModeNumHarmonics=1  ConsistencySolver=NEWTON_FTOL  IndexReductionMethod=DerivativeReplacement  DoDC=off  ResidualTolerance=1e-9  ConsistencyTolSource=GLOBAL  ConsistencyAbsTol=0.001  ConsistencyRelTol=0.001  ConsistencyTolFactor=0.001  UseLocalSolver=off  LocalSolverChoice=NE_BACKWARD_EULER_ADVANCER  ResolveIndetEquations=on  FunctionEvalNumThread=1  LocalSolverSampleTime=1  DoFixedCost=off  MaxNonlinIter=3  MaxModeIter=2  ComputeImpulses=off  ImpulseIterations=2  LinearAlgebra=Sparse  LinearAlgebraNumThread=0  EquationFormulation=NE_TIME_EF  DelaysMemoryBudget=1024  AutomaticFiltering=on  FilteringTimeConstant=0.001  PartitionStorageMethod=AS_NEEDED  PartitionMemoryBudget=1024  PartitionMethod=FAST
  T : PMIOPort  Side=Left
  wires:
  [Tamb] -> Simulink-PS Converter1/1
  connections:
  Simulink-PS Converter1/RConn1 -- Solver Configuration/RConn1 -- T/RConn1

== system batteryModel/Battery/Voltage Sensor ==
  PS-Simulink Converter : nesl_utility/PS-Simulink Converter  PhysicalDomain=network_engine_domain  SubClassName=ps_output  LeftPortType=input  RightPortType=output  PseudoPeriodic=off  Frequencies=[]  VectorFormat=1-D array  Unit=V  AffineConversion=off
  Voltage Sensor : fl_lib/Electrical/Electrical Sensors/Voltage Sensor
  + : PMIOPort  Side=Left
  - : PMIOPort  Port=2  Side=Right
  tag scope: V_load=global
  wires:
  PS-Simulink Converter/1 -> [V_load]
  connections:
  Voltage Sensor/RConn1 -- PS-Simulink Converter/LConn1
  +/RConn1 -- Voltage Sensor/LConn1
  -/RConn1 -- Voltage Sensor/RConn2

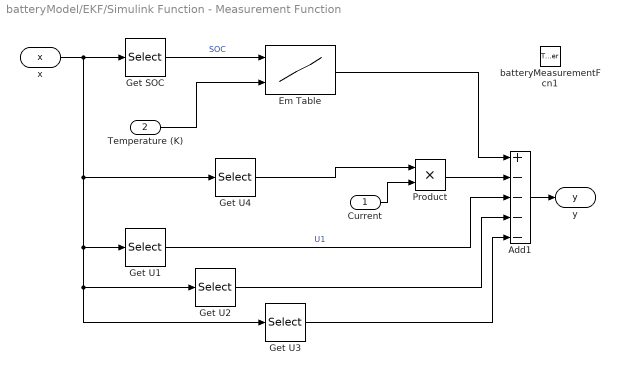
== system batteryModel/EKF/Simulink Function - Measurement Function ==
  Current : Inport
  Temperature (K) : Inport  Port=2
  batteryMeasurementFcn1 : TriggerPort  TriggerType=function-call  IsSimulinkFunction=on  FunctionName=batteryMeasurementFcn1  VariantControl=Variant
  Add1 : Sum  Inputs=+----
  Em Table : Lookup_n-D  BreakpointsForDimension1=Battery.SOC_LUT  BreakpointsForDimension2=Battery.Temperature_LUT  Table=Battery.Em_LUT  InternalRulePriority=Speed  RndMeth=Simplest
      settings: InputPortMap=u0,u1
  Get SOC : Selector  InputPortWidth=5  IndexOptions=Index vector (dialog)  Indices=[1]  OutputSizes=1
  Get U1 : Selector  InputPortWidth=5  IndexOptions=Index vector (dialog)  Indices=2  OutputSizes=1
  Get U2 : Selector  InputPortWidth=5  IndexOptions=Index vector (dialog)  Indices=3  OutputSizes=1
  Get U3 : Selector  InputPortWidth=5  IndexOptions=Index vector (dialog)  Indices=4  OutputSizes=1
  Get U4 : Selector  InputPortWidth=5  IndexOptions=Index vector (dialog)  Indices=5  OutputSizes=1
  Product : Product
  x : ArgIn  DisableCoverage=on  PortDimensions=5  ArgumentName=x
  y : ArgOut  DisableCoverage=on  ArgumentName=y
  wires:
  x/1 -> Get U4/1, Get U3/1, Get U2/1, Get U1/1, Get SOC/1
  Get SOC/1 -> Em Table/1  "SOC"
  Em Table/1 -> Add1/1
  Add1/1 -> y/1
  Temperature (K)/1 -> Em Table/2
  Get U4/1 -> Product/1
  Current/1 -> Product/2
  Product/1 -> Add1/2
  Get U1/1 -> Add1/3  "U1"
  Get U2/1 -> Add1/4
  Get U3/1 -> Add1/5

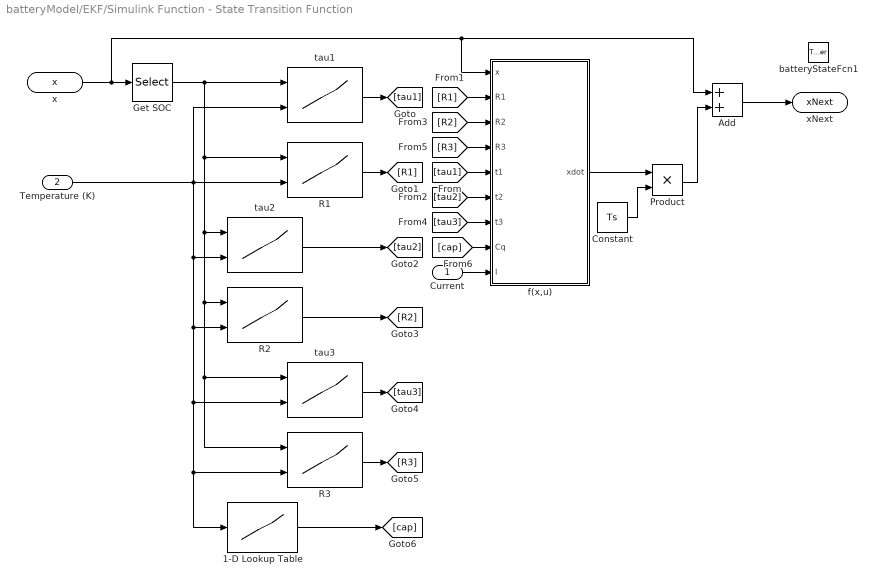
== system batteryModel/EKF/Simulink Function - State Transition Function ==
  Current : Inport
  Temperature (K) : Inport  Port=2
  batteryStateFcn1 : TriggerPort  TriggerType=function-call  IsSimulinkFunction=on  FunctionName=batteryStateFcn1  VariantControl=Variant
  1-D Lookup Table : Lookup_n-D  NumberOfTableDimensions=1  BreakpointsForDimension1=Battery.Temperature_LUT  Table=Battery.Capacity_LUT  InternalRulePriority=Speed  RndMeth=Simplest
  Add : Sum
  Constant : Constant  Value=Ts
  Get SOC : Selector  InputPortWidth=5  IndexOptions=Index vector (dialog)  Indices=1  OutputSizes=1
  Product : Product
  R1 : Lookup_n-D  BreakpointsForDimension1=Battery.SOC_LUT  BreakpointsForDimension2=Battery.Temperature_LUT  Table=Battery.R1_LUT  InternalRulePriority=Speed  RndMeth=Simplest
      settings: InputPortMap=u0,u1
  R2 : Lookup_n-D  BreakpointsForDimension1=Battery.SOC_LUT  BreakpointsForDimension2=Battery.Temperature_LUT  Table=Battery.R2_LUT  InternalRulePriority=Speed  RndMeth=Simplest
      settings: InputPortMap=u0,u1
  R3 : Lookup_n-D  BreakpointsForDimension1=Battery.SOC_LUT  BreakpointsForDimension2=Battery.Temperature_LUT  Table=Battery.R3_LUT  InternalRulePriority=Speed  RndMeth=Simplest
      settings: InputPortMap=u0,u1
  f(x,u) : MATLAB Function  TreatAsAtomicUnit=on
  tau1 : Lookup_n-D  BreakpointsForDimension1=Battery.SOC_LUT  BreakpointsForDimension2=Battery.Temperature_LUT  Table=Battery.t1_LUT  InternalRulePriority=Speed  RndMeth=Simplest
      settings: InputPortMap=u0,u1
  tau2 : Lookup_n-D  BreakpointsForDimension1=Battery.SOC_LUT  BreakpointsForDimension2=Battery.Temperature_LUT  Table=Battery.t2_LUT  InternalRulePriority=Speed  RndMeth=Simplest
      settings: InputPortMap=u0,u1
  tau3 : Lookup_n-D  BreakpointsForDimension1=Battery.SOC_LUT  BreakpointsForDimension2=Battery.Temperature_LUT  Table=Battery.t3_LUT  InternalRulePriority=Speed  RndMeth=Simplest
      settings: InputPortMap=u0,u1
  x : ArgIn  DisableCoverage=on  PortDimensions=5  ArgumentName=x
  xNext : ArgOut  DisableCoverage=on  PortDimensions=5  ArgumentName=xNext
  wires:
  x/1 -> f(x,u)/1(x), Add/1, Get SOC/1
  Add/1 -> xNext/1
  Temperature (K)/1 -> 1-D Lookup Table/1, R3/2, tau3/2, R2/2, tau2/2, R1/2, tau1/2
  Get SOC/1 -> R1/1, R3/1, tau3/1, R2/1, tau2/1, tau1/1
  Constant/1 -> Product/2
  f(x,u)/1(xdot) -> Product/1
  Product/1 -> Add/2
  tau1/1 -> [tau1]
  [tau1] -> f(x,u)/5(t1)
  R1/1 -> [R1]
  [R1] -> f(x,u)/2(R1)
  tau2/1 -> [tau2]
  [tau2] -> f(x,u)/6(t2)
  R2/1 -> [R2]
  [R2] -> f(x,u)/3(R2)
  R3/1 -> [R3]
  tau3/1 -> [tau3]
  [tau3] -> f(x,u)/7(t3)
  [R3] -> f(x,u)/4(R3)
  Current/1 -> f(x,u)/9(I)
  1-D Lookup Table/1 -> [cap]
  [cap] -> f(x,u)/8(Cq)

== system batteryModel/Function Fitting Neural Network/Layer 1 ==
  "p{1}" : Inport  PortDimensions=2
      mask Display: e = 0.06;c1 = [120 230 180]/255;c2 = ([120 230 180]+0)/(256+128);c3 = ([120 230 180]+128)/(256+128);patch([0 1 1 0],[0 0 1 1],c1);patch([0 1 1 1-e 1-e 0+e],[0 0 1 1-e 0+e 0+e],c2);patch([0 0 1 1-e 0+e 0+e],[0 1 1 1-e 1-e 0+e],c3);plot([0 1 1 0 0],[0 0 1 1 0]);
  Delays 1 : Subsystem
      mask Display: e = 0.06;c1 = [120 150 230]/255;c2 = ([120 150 230]+0)/383;c3 = ([120 150 230]+128)/383;patch([0 1 1 0],[0 0 1 1],c1);patch([0 1 1 1-e 1-e 0+e],[0 0 1 1-e 0+e 0+e],c2);patch([0 0 1 1-e 0+e 0+e],[0 1 1 1-e 1-e 0+e],c3);plot([0 1 1 0 0],[0 0 1 1 0]);disp('0');
  "IW{1,1}" : Subsystem
      mask Display: e = 0.06;c1 = [120 150 230]/255;c2 = ([120 150 230]+0)/383;c3 = ([120 150 230]+128)/383;patch([0 1 1 0],[0 0 1 1],c1);patch([0 1 1 1-e 1-e 0+e],[0 0 1 1-e 0+e 0+e],c2);patch([0 0 1 1-e 0+e 0+e],[0 1 1 1-e 1-e 0+e],c3);plot([0 1 1 0 0],[0 0 1 1 0]);disp('W');
  "b{1}" : Constant  Value=[6.1291160700631746038880010019056499004364013671875;-1.924970027675327433058782844454981386661529541015625;-5.80375123123512981493377083097584545612335205078125;5.8129730042097520481547689996659755706787109375;7.95940548155363725157940280041657388210296630859375;1.7954909112303247820108254018123261630535125732421875;-2.051073921165150526491061100387014448642730712890625;-6.48779633564738134055005502887070178985595703125;1.8958072543976267620990938667091540992259979248046875;0.0016263347402510892718285884228635040926747024059295654296875;0.498907047270881698342037680049543268978595733642578125;1.6020833473289066706257699479465372860431671142578125;0.470685936565122753361123386639519594609737396240234375;0.474537022679995590390689130799728445708751678466796875;5.54517016556591268994225174537859857082366943359375;3.10372333540804046236871727160178124904632568359375;5.62194556559681490881530407932586967945098876953125;-3.103279599172112934724054866819642484188079833984375;4.87036864836284877355865319259464740753173828125;5.96955689098831232541897406917996704578399658203125]
      mask Display: e = 0.06;c1 = [120 150 230]/255;c2 = ([120 150 230]+0)/383;c3 = ([120 150 230]+128)/383;patch([0 1 1 0],[0 0 1 1],c1);patch([0 1 1 1-e 1-e 0+e],[0 0 1 1-e 0+e 0+e],c2);patch([0 0 1 1-e 0+e 0+e],[0 1 1 1-e 1-e 0+e],c3);plot([0 1 1 0 0],[0 0 1 1 0]);disp('b');
  netsum : Sum  Inputs=2  InputSameDT=on  SaturateOnIntegerOverflow=on  OutDataTypeStr=Inherit: Same as first input
      mask Display: e = 0.06;c1 = [120 150 230]/255;c2 = ([120 150 230]+0)/383;c3 = ([120 150 230]+128)/383;patch([0 1 1 0],[0 0 1 1],c1);patch([0 1 1 1-e 1-e 0+e],[0 0 1 1-e 0+e 0+e],c2);patch([0 0 1 1-e 0+e 0+e],[0 1 1 1-e 1-e 0+e],c3);plot([0 1 1 0 0],[0 0 1 1 0]);disp('+');
  tansig : neural/Transfer Functions/tansig
  "a{1}" : Outport  InitialOutput=[0;0;0;0;0;0;0;0;0;0;0;0;0;0;0;0;0;0;0;0]
      mask Display: e = 0.06;c1 = [120 230 180]/255;c2 = ([120 230 180]+0)/(256+128);c3 = ([120 230 180]+128)/(256+128);patch([0 1 1 0],[0 0 1 1],c1);patch([0 1 1 1-e 1-e 0+e],[0 0 1 1-e 0+e 0+e],c2);patch([0 0 1 1-e 0+e 0+e],[0 1 1 1-e 1-e 0+e],c3);plot([0 1 1 0 0],[0 0 1 1 0]);
  wires:
  "p{1}"/1 -> Delays 1/1("p{1}")
  Delays 1/1("pd{1,1}") -> "IW{1,1}"/1("pd{1,1}")
  "IW{1,1}"/1("iz{1,1}") -> netsum/1
  "b{1}"/1 -> netsum/2
  netsum/1 -> tansig/1
  tansig/1 -> "a{1}"/1

== system batteryModel/Function Fitting Neural Network/Layer 2 ==
  "a{1} " : Inport  PortDimensions=20
      mask Display: e = 0.06;c1 = [120 230 180]/255;c2 = ([120 230 180]+0)/(256+128);c3 = ([120 230 180]+128)/(256+128);patch([0 1 1 0],[0 0 1 1],c1);patch([0 1 1 1-e 1-e 0+e],[0 0 1 1-e 0+e 0+e],c2);patch([0 0 1 1-e 0+e 0+e],[0 1 1 1-e 1-e 0+e],c3);plot([0 1 1 0 0],[0 0 1 1 0]);
  Delays 1 : Subsystem
      mask Display: e = 0.06;c1 = [120 150 230]/255;c2 = ([120 150 230]+0)/383;c3 = ([120 150 230]+128)/383;patch([0 1 1 0],[0 0 1 1],c1);patch([0 1 1 1-e 1-e 0+e],[0 0 1 1-e 0+e 0+e],c2);patch([0 0 1 1-e 0+e 0+e],[0 1 1 1-e 1-e 0+e],c3);plot([0 1 1 0 0],[0 0 1 1 0]);disp('0');
  "LW{2,1}" : Subsystem
      mask Display: e = 0.06;c1 = [120 150 230]/255;c2 = ([120 150 230]+0)/383;c3 = ([120 150 230]+128)/383;patch([0 1 1 0],[0 0 1 1],c1);patch([0 1 1 1-e 1-e 0+e],[0 0 1 1-e 0+e 0+e],c2);patch([0 0 1 1-e 0+e 0+e],[0 1 1 1-e 1-e 0+e],c3);plot([0 1 1 0 0],[0 0 1 1 0]);disp('W');
  "b{2}" : Constant  Value=0.0881216920410851367595483907280140556395053863525390625
      mask Display: e = 0.06;c1 = [120 150 230]/255;c2 = ([120 150 230]+0)/383;c3 = ([120 150 230]+128)/383;patch([0 1 1 0],[0 0 1 1],c1);patch([0 1 1 1-e 1-e 0+e],[0 0 1 1-e 0+e 0+e],c2);patch([0 0 1 1-e 0+e 0+e],[0 1 1 1-e 1-e 0+e],c3);plot([0 1 1 0 0],[0 0 1 1 0]);disp('b');
  netsum : Sum  Inputs=2  InputSameDT=on  SaturateOnIntegerOverflow=on  OutDataTypeStr=Inherit: Same as first input
      mask Display: e = 0.06;c1 = [120 150 230]/255;c2 = ([120 150 230]+0)/383;c3 = ([120 150 230]+128)/383;patch([0 1 1 0],[0 0 1 1],c1);patch([0 1 1 1-e 1-e 0+e],[0 0 1 1-e 0+e 0+e],c2);patch([0 0 1 1-e 0+e 0+e],[0 1 1 1-e 1-e 0+e],c3);plot([0 1 1 0 0],[0 0 1 1 0]);disp('+');
  purelin : neural/Transfer Functions/purelin
  "a{2}" : Outport  InitialOutput=0
      mask Display: e = 0.06;c1 = [120 230 180]/255;c2 = ([120 230 180]+0)/(256+128);c3 = ([120 230 180]+128)/(256+128);patch([0 1 1 0],[0 0 1 1],c1);patch([0 1 1 1-e 1-e 0+e],[0 0 1 1-e 0+e 0+e],c2);patch([0 0 1 1-e 0+e 0+e],[0 1 1 1-e 1-e 0+e],c3);plot([0 1 1 0 0],[0 0 1 1 0]);
  wires:
  "a{1} "/1 -> Delays 1/1("p{2}")
  Delays 1/1("pd{2,1}") -> "LW{2,1}"/1("ad{2,1}")
  "LW{2,1}"/1("lz{2,1}") -> netsum/1
  "b{2}"/1 -> netsum/2
  netsum/1 -> purelin/1
  purelin/1 -> "a{2}"/1

== system batteryModel/Function Fitting Neural Network/Process Input 1 ==
  x : Inport  PortDimensions=2
      mask Display: e = 0.06;c1 = [120 230 180]/255;c2 = ([120 230 180]+0)/(256+128);c3 = ([120 230 180]+128)/(256+128);patch([0 1 1 0],[0 0 1 1],c1);patch([0 1 1 1-e 1-e 0+e],[0 0 1 1-e 0+e 0+e],c2);patch([0 0 1 1-e 0+e 0+e],[0 1 1 1-e 1-e 0+e],c3);plot([0 1 1 0 0],[0 0 1 1 0]);
  mapminmax : neural/Processing Functions/mapminmax  xmin=[1.34608933921028106617256980826;-10.7374289544501255733166544815]  xmax=[4.26284564810847221849599009147;3.2018304176544631900469539687]  ymin=-1  ymax=1
  p : Outport  PortDimensions=2
      mask Display: e = 0.06;c1 = [120 230 180]/255;c2 = ([120 230 180]+0)/(256+128);c3 = ([120 230 180]+128)/(256+128);patch([0 1 1 0],[0 0 1 1],c1);patch([0 1 1 1-e 1-e 0+e],[0 0 1 1-e 0+e 0+e],c2);patch([0 0 1 1-e 0+e 0+e],[0 1 1 1-e 1-e 0+e],c3);plot([0 1 1 0 0],[0 0 1 1 0]);
  wires:
  x/1 -> mapminmax/1
  mapminmax/1 -> p/1
